simulink model "FIR_filter"  (R2020b)
settings: Solver=VariableStepAuto  StartTime=0.0  StopTime=100  RelTol=1e-3
settings Model: Creator=shraddha  LastModifiedBy=shraddha

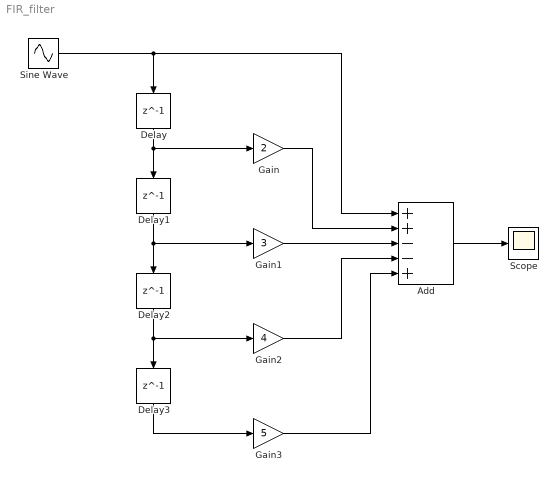
== system FIR_filter ==
  Add : Sum  Inputs=++--+
  Delay{,1..3} (4 alike) : Delay  DelayLength=1
  Gain : Gain  Gain=2
  Gain1 : Gain  Gain=3
  Gain2 : Gain  Gain=4
  Gain3 : Gain  Gain=5
  Scope : Scope
  Sine Wave : Sin  SampleTime=0
  wires:
  Delay/1 -> Gain/1, Delay1/1
  Delay1/1 -> Gain1/1, Delay2/1
  Delay2/1 -> Gain2/1, Delay3/1
  Delay3/1 -> Gain3/1
  Sine Wave/1 -> Delay/1, Add/1
  Gain/1 -> Add/2
  Gain1/1 -> Add/3
  Gain2/1 -> Add/4
  Gain3/1 -> Add/5
  Add/1 -> Scope/1
